simulink model "Budget"  (R2024a)
settings: Solver=VariableStepAuto  StartTime=0.0  StopTime=0  RelTol=1e-3
undefined symbols (not defined in the file): rational, rf, S, sparameters
libraries: simrfV2elements x5, simrfV2util1 x4, simrfV2systems x2, rfBudgetAnalyzer_lib x2, simrfV2sources1 x1
settings Model: Creator=rawas  LastModifiedBy=rawas

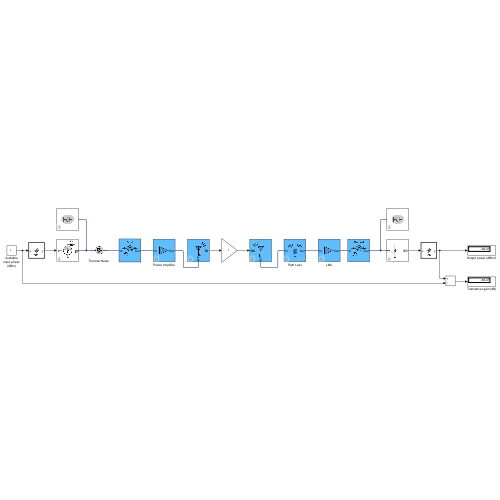
[thumbnail: Simulink's stored preview of the top-level diagram]
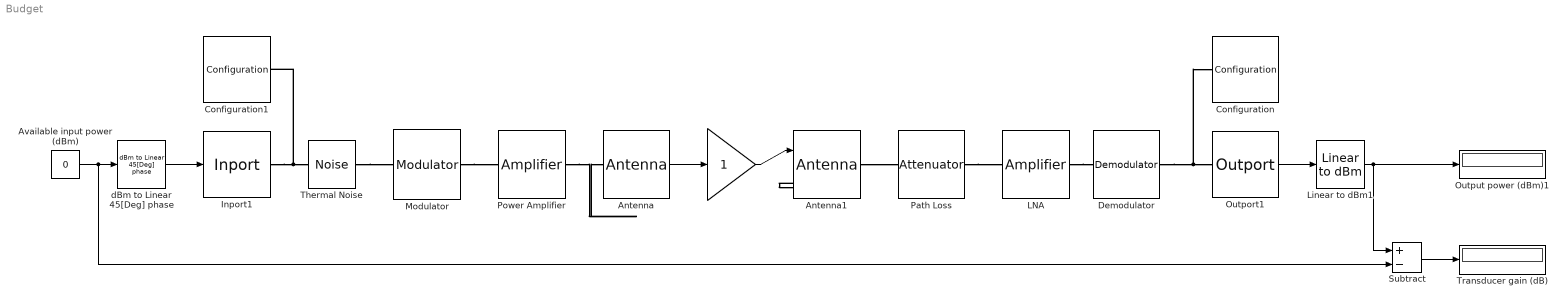
== system Budget ==
  " " : Gain
  Antenna : simrfV2elements/Antenna  CacheLevel=0  AntennaSource=Antenna object  PrevAppliedAntSource=Antenna object  Gr=2.12226563430722 dBi  Zin=80.7840831613671+2.57298129024611i  AntennaObj=TA  InputIncWave=off  OutputRadWave=on  CarrierFreqInc=2.1 GHz  rArr=[180 0] deg  CarrierFreqRad=5 GHz  rDep=[0 90] deg  AddNoise=on  InternalGrounding=on  SparamRepresentationImp=Time domain (rationalfit)  FitTolImp=-40  AutoImpulseLengthImp=on  ImpulseLengthImp=1e-10 s
  Antenna1 : simrfV2elements/Antenna  CacheLevel=0  AntennaSource=Antenna object  PrevAppliedAntSource=Antenna object  Gr=2.12226563430722 dBi  Zin=80.7841+2.57298i  AntennaObj=RA  InputIncWave=on  OutputRadWave=off  CarrierFreqInc=5 GHz  rArr=[180 0] deg  CarrierFreqRad=2.1 GHz  rDep=[0 0] deg  AddNoise=on  InternalGrounding=on  SparamRepresentationImp=Time domain (rationalfit)  FitTolImp=-40  AutoImpulseLengthImp=on  ImpulseLengthImp=1e-10 s
  Available input power (dBm) : Constant  Value=0
  Configuration : simrfV2util1/Configuration  AutoFreq=on  Tones=[] Hz  Harmonics=[]  NormalizeCarrierPower=on  SolverType=Auto  UseCCode=on  StepSize=(1/100000000)/8 s  AddNoise=on  defaultRNG=on  Seed=0  Temperature=290.0 K  SolverDelFlag=0  AbsTol=1e-6  RelTol=1e-3  MaxIter=10  ErrorEstimationType=2-norm over all variables  EnableInterpFilter=on  HiddenFIRfilterControllerParam=on  SmallSignalApprox=off  AllSimFreqs=on  SimFreqs=[] Hz  SimFreqsInternal=[]  SamplesPerFrame=1
  Configuration1 : simrfV2util1/Configuration  AutoFreq=on  Tones=[] Hz  Harmonics=[]  NormalizeCarrierPower=on  SolverType=Auto  UseCCode=on  StepSize=(1/100000000)/8 s  AddNoise=on  defaultRNG=on  Seed=0  Temperature=290.0 K  SolverDelFlag=0  AbsTol=1e-6  RelTol=1e-3  MaxIter=10  ErrorEstimationType=2-norm over all variables  EnableInterpFilter=on  HiddenFIRfilterControllerParam=on  SmallSignalApprox=off  AllSimFreqs=on  SimFreqs=[] Hz  SimFreqsInternal=[]  SamplesPerFrame=1
  Demodulator : simrfV2systems/Demodulator  classname=rfdemod  Source_linear_gain=Available power gain  linear_gain=15 dB  Poly_Coeffs=[0 1]  LOFreq=4.992 GHz  Zin=50  Zout=50  AddIRFilter=on  AddCSFilter=on  InternalGrounding=on  ForceNextInit=off  Source_Poly=Even and odd order  IPType=Output  IP2=Inf dBm  IP3=30 dBm  P1dB=inf dBm  Psat=inf dBm  Gcomp=inf dBm  NF=7.5  Isolation=inf dB  AddPhaseNoise=off  PhaseNoiseOffset=1  PhaseNoiseLevel=-Inf  AutoImpulseLengthPN=on  ImpulseLengthPN=1e-10  ImpulseLength_unitPN=s  DesignMethodIR=Ideal  ResponseTypeIR=Highpass  ImplementationIR=LC Tee  ImplementationIdealIR=Constant per carrier  ImplementationRationalIR=Transfer function  UseFilterOrderIR=on  FilterOrderIR=3  PassFreq_lpIR=5.05  PassFreq_lp_unitIR=GHz  PassFreq_hpIR=4.984000001  PassFreq_hp_unitIR=GHz  PassFreq_bpIR=[4.984000001 5.05]  PassFreq_bp_unitIR=GHz  PassFreq_bsIR=[4.933999999 4.984000001]  PassFreq_bs_unitIR=GHz  PassAttenIR=10*log10(2)  StopFreq_lpIR=5.050000001  StopFreq_lp_unitIR=GHz  StopFreq_hpIR=4.984  StopFreq_hp_unitIR=GHz  StopFreq_bpIR=[4.984 5.050000001]  StopFreq_bp_unitIR=GHz  StopFreq_bsIR=[4.934 4.984]  StopFreq_bs_unitIR=GHz  StopAttenIR=40  RsrcIR=50  RloadIR=50  AutoImpulseLengthIR=on  ImpulseLengthIR=1e-10  ImpulseLength_unitIR=s  DesignMethodCS=Ideal  ResponseTypeCS=Lowpass  ImplementationCS=LC Tee  ImplementationIdealCS=Constant per carrier  ImplementationRationalCS=Transfer function  UseFilterOrderCS=on  FilterOrderCS=3  PassFreq_lpCS=58  PassFreq_lp_unitCS=MHz  PassFreq_hpCS=0  PassFreq_hp_unitCS=Hz  PassFreq_bpCS=[0 58]  PassFreq_bp_unitCS=MHz  PassFreq_bsCS=[9.941999999 10.042000001]  PassFreq_bs_unitCS=GHz  PassAttenCS=10*log10(2)  StopFreq_lpCS=58.000001  StopFreq_lp_unitCS=MHz  StopFreq_hpCS=0  StopFreq_hp_unitCS=Hz  StopFreq_bpCS=[0 58.000001]  StopFreq_bp_unitCS=MHz  StopFreq_bsCS=[9.942 10.042]  StopFreq_bs_unitCS=GHz  StopAttenCS=40  RsrcCS=50  RloadCS=50  AutoImpulseLengthCS=on  ImpulseLengthCS=1e-10  ImpulseLength_unitCS=s
  Inport1 : simrfV2util1/Inport  SimulinkInputSignalType=Power  CarrierFreq=8 MHz  ZS=50  UseSqWave=off  NumCoeff=10  Bias=0  DutyCyc=50  InternalGrounding=on
  LNA : simrfV2elements/Amplifier  classname=amplifier  DataSource=Data file  File=unitygain.s2p  isNetworkObj=off  NetworkObject=sparameters('default.s2p')  Paramtype=S-parameters  Sparam=[0 0;1 0]  SparamFreq=1e9 Hz  SparamZ0=50  isRationalObj=off  RationalObject=rational('default.s2p')  Residues=0  Poles=0  DF={0 0; 1 0}  Source_linear_gain=Available power gain  linear_gain=30 dB  AmAmAmPmTable=[-25,5,-1;-10,20,-2;0,27,5;5,28,12]  Zin=50  Zout=50  Source_Poly=Even and odd order  Poly_Coeffs=[0 1]  IPType=Output  IP2=Inf dBm  IP3=32.5 dBm  P1dB=inf dBm  Psat=inf dBm  Gcomp=inf dBm  InternalGrounding=on  SourceFreq=Extracted from data source  PlotFreq=[1e9:1e6:3e9] Hz  PlotType=X-Y plane  YParam1=S(1,1)  YFormat1=Magnitude (dB)  YParam2=None  YFormat2=Magnitude (dB)  YOption=Linear  XOption=Linear  SparamRepresentation=Time domain (rationalfit)  FitTol=-40  FitOpt=Fit individually  MaxPoles=48  AutoImpulseLength=on  ImpulseLength=1e-10 s  MagModeling=off  AddNoise=on  NoiseType=Noise figure  NoiseDist=White  NF=0.56  MinNF=0  Gopt=0  RN=0  CarrierFreq=0 Hz  NoiseAutoImpulseLength=on  NoiseImpulseLength=1e-10 s  ConstS21NL=off  OpFreq=1 GHz  SetOpFreqAsMaxS21=off
  Linear to dBm1 : rfBudgetAnalyzer_lib/Linear to dBm  SystemSampleTime=-1  VariantActivationTime=update diagram  AllowFlexibleInterface=on  Latency=0  AutoFrameSizeCalculation=off
  Modulator : simrfV2systems/Modulator  classname=rfmod  Source_linear_gain=Available power gain  linear_gain=16 dB  Poly_Coeffs=[0 1]  LOFreq=4.992 GHz  Zin=50  Zout=50  AddIRFilter=on  AddCSFilter=on  InternalGrounding=on  ForceNextInit=off  Source_Poly=Even and odd order  IPType=Output  IP2=Inf dBm  IP3=35 dBm  P1dB=inf dBm  Psat=inf dBm  Gcomp=inf dBm  NF=7.5  Isolation=inf dB  AddPhaseNoise=off  PhaseNoiseOffset=1  PhaseNoiseLevel=-Inf  AutoImpulseLengthPN=on  ImpulseLengthPN=1e-10  ImpulseLength_unitPN=s  DesignMethodIR=Ideal  ResponseTypeIR=Lowpass  ImplementationIR=LC Tee  ImplementationIdealIR=Constant per carrier  ImplementationRationalIR=Transfer function  UseFilterOrderIR=on  FilterOrderIR=3  PassFreq_lpIR=58  PassFreq_lp_unitIR=MHz  PassFreq_hpIR=0  PassFreq_hp_unitIR=Hz  PassFreq_bpIR=[0 58]  PassFreq_bp_unitIR=MHz  PassFreq_bsIR=[9.941999999 10.042000001]  PassFreq_bs_unitIR=GHz  PassAttenIR=10*log10(2)  StopFreq_lpIR=58.000001  StopFreq_lp_unitIR=MHz  StopFreq_hpIR=0  StopFreq_hp_unitIR=Hz  StopFreq_bpIR=[0 58.000001]  StopFreq_bp_unitIR=MHz  StopFreq_bsIR=[9.942 10.042]  StopFreq_bs_unitIR=GHz  StopAttenIR=40  RsrcIR=50  RloadIR=50  AutoImpulseLengthIR=on  ImpulseLengthIR=1e-10  ImpulseLength_unitIR=s  DesignMethodCS=Ideal  ResponseTypeCS=Highpass  ImplementationCS=LC Tee  ImplementationIdealCS=Constant per carrier  ImplementationRationalCS=Transfer function  UseFilterOrderCS=on  FilterOrderCS=3  PassFreq_lpCS=5.05  PassFreq_lp_unitCS=GHz  PassFreq_hpCS=4.984000001  PassFreq_hp_unitCS=GHz  PassFreq_bpCS=[4.984000001 5.05]  PassFreq_bp_unitCS=GHz  PassFreq_bsCS=[4.933999999 4.984000001]  PassFreq_bs_unitCS=GHz  PassAttenCS=10*log10(2)  StopFreq_lpCS=5.050000001  StopFreq_lp_unitCS=GHz  StopFreq_hpCS=4.984  StopFreq_hp_unitCS=GHz  StopFreq_bpCS=[4.984 5.050000001]  StopFreq_bp_unitCS=GHz  StopFreq_bsCS=[4.934 4.984]  StopFreq_bs_unitCS=GHz  StopAttenCS=40  RsrcCS=50  RloadCS=50  AutoImpulseLengthCS=on  ImpulseLengthCS=1e-10  ImpulseLength_unitCS=s
  Outport1 : simrfV2util1/Outport  SensorType=Power  OutputFormat=Complex Baseband  CarrierFreq=8 MHz  ZL=50  InternalGrounding=on  StepSize=1e-6 s  AutoStep=on  HalfPolyphaseLength=12
  Output power (dBm)1 : Display
  Path Loss : simrfV2elements/Attenuator  classname=attenuator  Att=PL  Zin=50  Zout=50  AddNoise=on  InternalGrounding=on
  Power Amplifier : simrfV2elements/Amplifier  classname=amplifier  DataSource=Data file  File=unitygain.s2p  isNetworkObj=off  NetworkObject=sparameters('default.s2p')  Paramtype=S-parameters  Sparam=[0 0;1 0]  SparamFreq=1e9 Hz  SparamZ0=50  isRationalObj=off  RationalObject=rational('default.s2p')  Residues=0  Poles=0  DF={0 0; 1 0}  Source_linear_gain=Available power gain  linear_gain=15 dB  AmAmAmPmTable=[-25,5,-1;-10,20,-2;0,27,5;5,28,12]  Zin=50  Zout=50  Source_Poly=Even and odd order  Poly_Coeffs=[0 1]  IPType=Output  IP2=Inf dBm  IP3=40 dBm  P1dB=inf dBm  Psat=inf dBm  Gcomp=inf dBm  InternalGrounding=on  SourceFreq=Extracted from data source  PlotFreq=[1e9:1e6:3e9] Hz  PlotType=X-Y plane  YParam1=S(1,1)  YFormat1=Magnitude (dB)  YParam2=None  YFormat2=Magnitude (dB)  YOption=Linear  XOption=Linear  SparamRepresentation=Time domain (rationalfit)  FitTol=-40  FitOpt=Fit individually  MaxPoles=48  AutoImpulseLength=on  ImpulseLength=1e-10 s  MagModeling=off  AddNoise=on  NoiseType=Noise figure  NoiseDist=White  NF=7.5  MinNF=0  Gopt=0  RN=0  CarrierFreq=0 Hz  NoiseAutoImpulseLength=on  NoiseImpulseLength=1e-10 s  ConstS21NL=off  OpFreq=1 GHz  SetOpFreqAsMaxS21=off
  Subtract : Sum  Inputs=+-
  Thermal Noise : simrfV2sources1/Noise  SimulinkInputSignalType=Ideal voltage  NoiseType=White  NoisePSD=4*rf.physconst('Boltzmann')*290*50  CarrierFreq=0 Hz  AutoImpulseLength=on  ImpulseLength=1e-10 s  InternalGrounding=off
  Transducer gain (dB) : Display
  dBm to Linear 45[Deg] phase : rfBudgetAnalyzer_lib/dBm to Linear 45[Deg] phase  SystemSampleTime=-1  VariantActivationTime=update diagram  AllowFlexibleInterface=on  Latency=0  AutoFrameSizeCalculation=off
  wires:
  Available input power (dBm)/1 -> dBm to Linear 45[Deg] phase/1, Subtract/2
  dBm to Linear 45[Deg] phase/1 -> Inport1/1
  Antenna/1 -> " "/1
  " "/1 -> Antenna1/1
  Outport1/1 -> Linear to dBm1/1
  Linear to dBm1/1 -> Output power (dBm)1/1, Subtract/1
  Subtract/1 -> Transducer gain (dB)/1
  connections:
  Configuration1/LConn1 -- Inport1/RConn1 -- Thermal Noise/RConn1
  Thermal Noise/LConn1 -- Modulator/LConn1
  Modulator/RConn1 -- Power Amplifier/LConn1
  Power Amplifier/RConn1 -- Antenna/LConn1
  Antenna1/LConn1 -- Path Loss/LConn1
  Path Loss/RConn1 -- LNA/LConn1
  LNA/RConn1 -- Demodulator/LConn1
  Demodulator/RConn1 -- Configuration/LConn1 -- Outport1/LConn1
